simulink model "EsamblajeCohete2_0"  (R2023a)
settings: Solver=VariableStepAuto  StartTime=0.0  StopTime=15  RelTol=1e-3
model workspace: external: MATLAB File C:\Users\SEBASTIANDIAZPABON\OneDrive - Universidad Santo Tomás Bucaramanga\USTA\Semillero Cohete\Cohete Matlab 2.0\EsamblajeCohete2_0_DataFile.m (data not in the file)
undefined symbols (not defined in the file): smiData, X, Y, Z
libraries: sm_lib x355, nesl_utility x10, fuzblock x4, simulink x2
(part 7 of 7)

== system EsamblajeCohete2_0/Cohete/Assembly_4_RIGID/Rotor_Cover_1_RIGID ==
  ReferenceFrame : sm_lib/Frames and Transforms/Reference Frame
  Solid : sm_lib/Body Elements/File Solid  ExtGeomFileName=Rotor Cover_Default_sldprt.STEP  UnitType=FromFile  ExtGeomFileUnits=m  StepReaderType=HEX  ExportConvexHullGeometry=off  InertiaType=Custom  Mass=smiData.Solid(11).mass  MassUnits=kg  CenterOfMass=smiData.Solid(11).CoM  CenterOfMassUnits=mm  MomentsOfInertia=smiData.Solid(11).MoI  MomentsOfInertiaUnits=kg*mm^2  ProductsOfInertia=smiData.Solid(11).PoI  ProductsOfInertiaUnits=kg*mm^2  BasedOnType=DensityFromFile  Density=1000  DensityUnits=kg/m^3  DoExposeReferenceFrame=on  SerializedFrames=<Frames/>  GraphicType=FromGeometry  MarkerShape=Sphere  MarkerSize=10  GraphicVisPropType=SimpleVisualProperties  GraphicDiffuseColor=smiData.Solid(11).color  GraphicSpecularColor=[0.5 0.5 0.5 1.0]  GraphicAmbientColor=[0.15 0.15 0.15 1.0]  GraphicEmissiveColor=[0.0 0.0 0.0 1.0]  GraphicShininess=75  GraphicOpacity=smiData.Solid(11).opacity
  F : PMIOPort  Side=Left
  connections:
  Solid/RConn1 -- ReferenceFrame/RConn1 -- F/RConn1

== system EsamblajeCohete2_0/Cohete/Assembly_4_RIGID/Stopper_Screw_1_RIGID ==
  ReferenceFrame : sm_lib/Frames and Transforms/Reference Frame
  Solid : sm_lib/Body Elements/File Solid  ExtGeomFileName=Stopper Screw_Default_sldprt.STEP  UnitType=FromFile  ExtGeomFileUnits=m  StepReaderType=HEX  ExportConvexHullGeometry=off  InertiaType=Custom  Mass=smiData.Solid(12).mass  MassUnits=kg  CenterOfMass=smiData.Solid(12).CoM  CenterOfMassUnits=mm  MomentsOfInertia=smiData.Solid(12).MoI  MomentsOfInertiaUnits=kg*mm^2  ProductsOfInertia=smiData.Solid(12).PoI  ProductsOfInertiaUnits=kg*mm^2  BasedOnType=DensityFromFile  Density=1000  DensityUnits=kg/m^3  DoExposeReferenceFrame=on  SerializedFrames=<Frames/>  GraphicType=FromGeometry  MarkerShape=Sphere  MarkerSize=10  GraphicVisPropType=SimpleVisualProperties  GraphicDiffuseColor=smiData.Solid(12).color  GraphicSpecularColor=[0.5 0.5 0.5 1.0]  GraphicAmbientColor=[0.15 0.15 0.15 1.0]  GraphicEmissiveColor=[0.0 0.0 0.0 1.0]  GraphicShininess=75  GraphicOpacity=smiData.Solid(12).opacity
  F : PMIOPort  Side=Left
  connections:
  Solid/RConn1 -- ReferenceFrame/RConn1 -- F/RConn1

== system EsamblajeCohete2_0/Cohete/Assembly_4_RIGID/e_ring_external_retaining_ring_wti_4_RIGID ==
  ReferenceFrame : sm_lib/Frames and Transforms/Reference Frame
  Solid : sm_lib/Body Elements/File Solid  ExtGeomFileName=e-ring external retaining ring_wti_Truarc X5133-14 - S0.14_sldprt.STEP  UnitType=FromFile  ExtGeomFileUnits=m  StepReaderType=HEX  ExportConvexHullGeometry=off  InertiaType=Custom  Mass=smiData.Solid(10).mass  MassUnits=kg  CenterOfMass=smiData.Solid(10).CoM  CenterOfMassUnits=in  MomentsOfInertia=smiData.Solid(10).MoI  MomentsOfInertiaUnits=kg*in^2  ProductsOfInertia=smiData.Solid(10).PoI  ProductsOfInertiaUnits=kg*in^2  BasedOnType=DensityFromFile  Density=1000  DensityUnits=kg/m^3  DoExposeReferenceFrame=on  SerializedFrames=<Frames/>  GraphicType=FromGeometry  MarkerShape=Sphere  MarkerSize=10  GraphicVisPropType=SimpleVisualProperties  GraphicDiffuseColor=smiData.Solid(10).color  GraphicSpecularColor=[0.5 0.5 0.5 1.0]  GraphicAmbientColor=[0.15 0.15 0.15 1.0]  GraphicEmissiveColor=[0.0 0.0 0.0 1.0]  GraphicShininess=75  GraphicOpacity=smiData.Solid(10).opacity
  F : PMIOPort  Side=Left
  connections:
  Solid/RConn1 -- ReferenceFrame/RConn1 -- F/RConn1

== system EsamblajeCohete2_0/Cohete/Assembly_4_RIGID/instrument_ball_bearing_68_iso_1_RIGID ==
  ReferenceFrame : sm_lib/Frames and Transforms/Reference Frame
  Solid : sm_lib/Body Elements/File Solid  ExtGeomFileName=instrument ball bearing_68_iso_ISO 1224 - 390308 - R-8-DE-NC-8_68_sldprt.STEP  UnitType=FromFile  ExtGeomFileUnits=m  StepReaderType=HEX  ExportConvexHullGeometry=off  InertiaType=Custom  Mass=smiData.Solid(14).mass  MassUnits=kg  CenterOfMass=smiData.Solid(14).CoM  CenterOfMassUnits=mm  MomentsOfInertia=smiData.Solid(14).MoI  MomentsOfInertiaUnits=kg*mm^2  ProductsOfInertia=smiData.Solid(14).PoI  ProductsOfInertiaUnits=kg*mm^2  BasedOnType=DensityFromFile  Density=1000  DensityUnits=kg/m^3  DoExposeReferenceFrame=on  SerializedFrames=<Frames/>  GraphicType=FromGeometry  MarkerShape=Sphere  MarkerSize=10  GraphicVisPropType=SimpleVisualProperties  GraphicDiffuseColor=smiData.Solid(14).color  GraphicSpecularColor=[0.5 0.5 0.5 1.0]  GraphicAmbientColor=[0.15 0.15 0.15 1.0]  GraphicEmissiveColor=[0.0 0.0 0.0 1.0]  GraphicShininess=75  GraphicOpacity=smiData.Solid(14).opacity
  F : PMIOPort  Side=Left
  connections:
  Solid/RConn1 -- ReferenceFrame/RConn1 -- F/RConn1

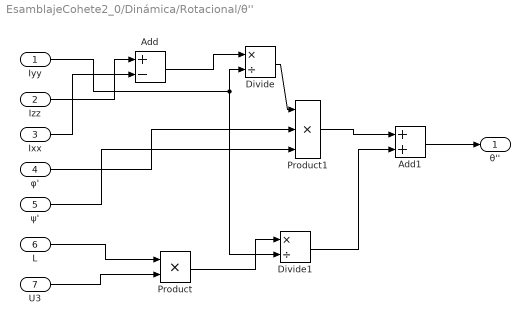
== system EsamblajeCohete2_0/Dinámica/Rotacional/θ'' ==
  Iyy : Inport
  Izz : Inport  Port=2
  Ixx : Inport  Port=3
  φ' : Inport  Port=4
  ψ' : Inport  Port=5
  L : Inport  Port=6
  U3 : Inport  Port=7
  Add : Sum  Inputs=+-
  Add1 : Sum
  Divide : Product  Inputs=*/
  Divide1 : Product  Inputs=*/
  Product : Product
  Product1 : Product  Inputs=3
  θ'' : Outport
  wires:
  Add/1 -> Divide/1
  Divide/1 -> Product1/1
  Product/1 -> Divide1/1
  Product1/1 -> Add1/1
  Divide1/1 -> Add1/2
  Add1/1 -> θ''/1
  Iyy/1 -> Divide1/2, Divide/2
  Izz/1 -> Add/1
  Ixx/1 -> Add/2
  φ'/1 -> Product1/2
  ψ'/1 -> Product1/3
  L/1 -> Product/1
  U3/1 -> Product/2

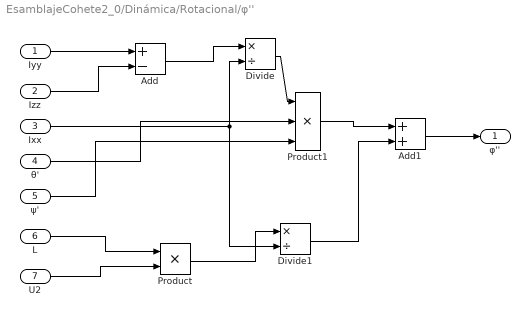
== system EsamblajeCohete2_0/Dinámica/Rotacional/φ'' ==
  Iyy : Inport
  Izz : Inport  Port=2
  Ixx : Inport  Port=3
  θ' : Inport  Port=4
  ψ' : Inport  Port=5
  L : Inport  Port=6
  U2 : Inport  Port=7
  Add : Sum  Inputs=+-
  Add1 : Sum
  Divide : Product  Inputs=*/
  Divide1 : Product  Inputs=*/
  Product : Product
  Product1 : Product  Inputs=3
  φ'' : Outport
  wires:
  Iyy/1 -> Add/1
  Izz/1 -> Add/2
  Add/1 -> Divide/1
  Ixx/1 -> Divide1/2, Divide/2
  Divide/1 -> Product1/1
  θ'/1 -> Product1/2
  ψ'/1 -> Product1/3
  L/1 -> Product/1
  U2/1 -> Product/2
  Product/1 -> Divide1/1
  Product1/1 -> Add1/1
  Divide1/1 -> Add1/2
  Add1/1 -> φ''/1

== system EsamblajeCohete2_0/Dinámica/Rotacional/ψ'' ==
  Iyy : Inport
  Izz : Inport  Port=2
  Ixx : Inport  Port=3
  φ' : Inport  Port=4
  θ' : Inport  Port=5
  L : Inport  Port=6
  U4 : Inport  Port=7
  Add : Sum  Inputs=+-
  Add1 : Sum
  Divide : Product  Inputs=*/
  Divide1 : Product  Inputs=*/
  Product : Product
  Product1 : Product  Inputs=3
  ψ'' : Outport
  wires:
  Add/1 -> Divide/1
  Divide/1 -> Product1/1
  Product/1 -> Divide1/1
  Product1/1 -> Add1/1
  Divide1/1 -> Add1/2
  Add1/1 -> ψ''/1
  Iyy/1 -> Add/2
  Ixx/1 -> Add/1
  Izz/1 -> Divide1/2, Divide/2
  φ'/1 -> Product1/2
  θ'/1 -> Product1/3
  L/1 -> Product/1
  U4/1 -> Product/2
